simulink model "Cinetique_robot"  (R2021b)
settings: Solver=VariableStepAuto  StartTime=0.0  StopTime=10.0  RelTol=1e-3
settings Model: DataDictionary=RobotModel.sldd  EnableAccessToBaseWorkspace=off  Creator=hugo  LastModifiedBy=hugo
settings SolverCC: AlgebraicLoopSolver=TrustRegion
settings DataIOCC: SaveOutput=off  SaveTime=off  ReturnWorkspaceOutputs=off
settings DebuggingCC: SFMachineParentedDataDiag=warning  ArithmeticOperatorsInVariantConditions=warning
settings SFSimCC: SimUseLocalCustomCode=off  CustomCodeUndefinedFunction=UseInterfaceOnly
settings RTWCC: RTWUseLocalCustomCode=off

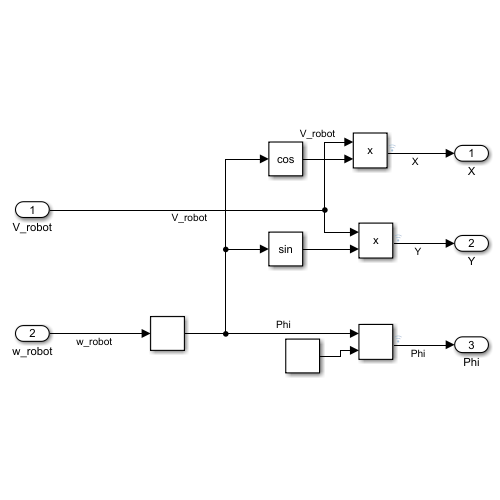
[thumbnail: Simulink's stored preview of the top-level diagram]
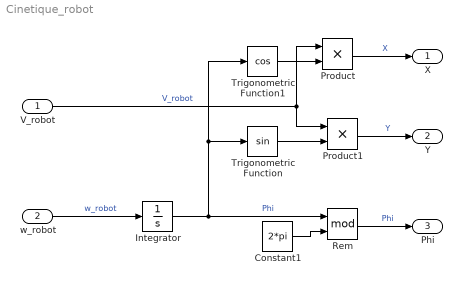
== system Cinetique_robot ==
  V_robot : Inport  OutDataTypeStr=double  PortDimensions=1  SampleTime=0
  w_robot : Inport  Port=2  OutDataTypeStr=double  PortDimensions=1  SampleTime=0
  Constant1 : Constant  Value=2*pi
  Integrator : Integrator  ContinuousStateAttributes='robot_angle'
  Product : Product
  Product1 : Product
  Rem : Math  Operator=mod  SignedPower=on  SaturateOnIntegerOverflow=on
  Trigonometric Function : Trigonometry
  Trigonometric Function1 : Trigonometry  Operator=cos
  X : Outport  OutDataTypeStr=double  PortDimensions=1  SampleTime=0  VectorParamsAs1DForOutWhenUnconnected=off
  Y : Outport  Port=2  OutDataTypeStr=double  PortDimensions=1  SampleTime=0  VectorParamsAs1DForOutWhenUnconnected=off
  Phi : Outport  Port=3  OutDataTypeStr=double  PortDimensions=1  SampleTime=0  VectorParamsAs1DForOutWhenUnconnected=off
  wires:
  Rem/1 -> Phi/1  "Phi"
  Constant1/1 -> Rem/2
  Product1/1 -> Y/1  "Y"
  Trigonometric Function/1 -> Product1/2
  Trigonometric Function1/1 -> Product/2
  Product/1 -> X/1  "X"
  Integrator/1 -> Rem/1, Trigonometric Function1/1, Trigonometric Function/1  "Phi"
  w_robot/1 -> Integrator/1  "w_robot"
  V_robot/1 -> Product/1, Product1/1  "V_robot"
